simulink model "projesim1"  (R2019a)
settings: Solver=VariableStepAuto  StartTime=0.0  StopTime=10.0  RelTol=1e-3
values from neighbouring files (symbols this model uses):
  A = [ 0 1 0 0 ; 0 0 1 0 ; 0 0 0 1 ; 0 0 (-Ks * (M1+M2)/M1 * M2) 0]    [HANDECODE.m]
  C = [1 0 0 0]    [HANDECODE.m]
settings Model: Creator=handeyildirim  LastModifiedBy=handeyildirim

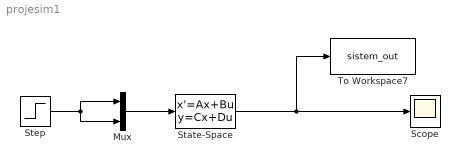
== system projesim1 ==
  Mux : Mux  Inputs=2
  Scope : Scope
  State-Space : StateSpace  A=A  B=[1 1; 1 1; 1 1; 1 1]  C=C  D=[0 0]  InitialCondition=[0]
  Step : Step  SampleTime=0
  To Workspace7 : ToWorkspace  VariableName=sistem_out  SaveFormat=Timeseries  SampleTime=-1
  wires:
  Mux/1 -> State-Space/1
  Step/1 -> Mux/2, Mux/1
  State-Space/1 -> To Workspace7/1, Scope/1
